simulink model "simu"  (R2023b)
settings: Solver=ode15s  StartTime=0.0  StopTime=20  RelTol=1e-4
values from neighbouring files (symbols this model uses):
  Bm = .015    (= 0.015)    [example_1.m]    (also in myStateTransitionFcn.m)
  g = 9.8    [example_1.m]    (also in myStateTransitionFcn.m)
  J = 4e-4    (= 0.0004)    [example_1.m]    (also in myStateTransitionFcn.m)
  Jl = 4e-4    (= 0.0004)    [example_1.m]    (also in myStateTransitionFcn.m)
  Jm = 4e-4    (= 0.0004)    [example_1.m]    (also in myStateTransitionFcn.m)
  k = .8    (= 0.8)    [example_1.m]    (also in myStateTransitionFcn.m)
  l = .3    (= 0.3)    [example_1.m]    (also in myStateTransitionFcn.m)
  m = .3    (= 0.3)    [example_1.m]    (also in myStateTransitionFcn.m)
  static_gain = inv(C*inv(-A+B*K)*B)    [example_1.m]
  x_est_initial = [pi/2;0;pi/2;0]    [example_1.m]
undefined symbols (not defined in the file or in its folder): beta, K
settings Model: Creator=Douglas  LastModifiedBy=Douglas

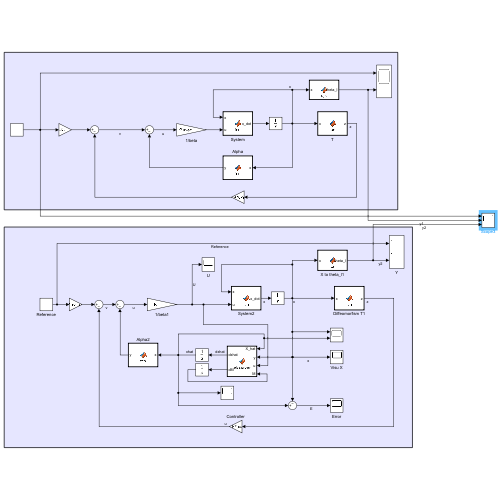
[thumbnail: Simulink's stored preview of the top-level diagram]
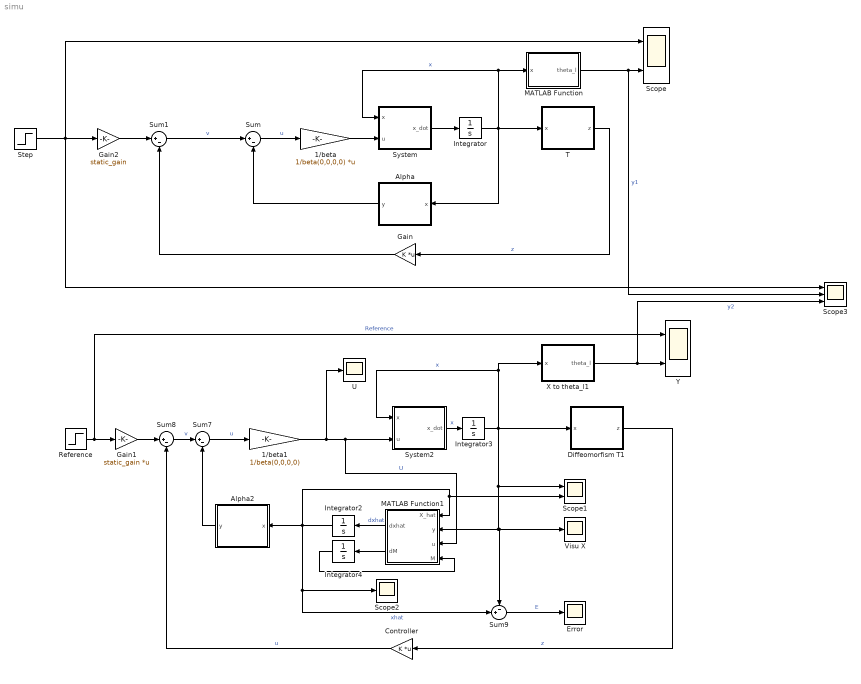
== system simu ==
  1/beta : Gain  Gain=1/beta(0,0,0,0)  Multiplication=Matrix(K*u) (u vector)
  1/beta1 : Gain  Gain=1/beta(0,0,0,0)
  Alpha : MATLAB Function  TreatAsAtomicUnit=on
  Alpha2 : MATLAB Function  TreatAsAtomicUnit=on
  Controller : Gain  Gain=K  Multiplication=Matrix(K*u) (u vector)
  Diffeomorfism T1 : MATLAB Function  TreatAsAtomicUnit=on
  Error : Scope
  Gain : Gain  Gain=K  Multiplication=Matrix(K*u) (u vector)
  Gain1 : Gain  Gain=static_gain  Multiplication=Matrix(K*u) (u vector)
  Gain2 : Gain  Gain=static_gain
  Integrator : Integrator  InitialCondition=x_est_initial
  Integrator2 : Integrator  InitialCondition=x_est_initial
  Integrator3 : Integrator  InitialCondition=x_est_initial
  Integrator4 : Integrator  InitialCondition=zeros(4,4)
  MATLAB Function : MATLAB Function  TreatAsAtomicUnit=on
  MATLAB Function1 : MATLAB Function  TreatAsAtomicUnit=on
  Reference : Step  Time=10  After=0.3  SampleTime=0
  Scope : Scope  NumInputPorts=2
  Scope1 : Scope  NumInputPorts=2
  Scope2 : Scope
  Scope3 : Scope  NumInputPorts=3
  Step : Step  Time=10  After=0.3  SampleTime=0
  Sum{,1,7..8} (4 alike) : Sum  Inputs=|+-
  Sum9 : Sum  Inputs=-+|
  System : MATLAB Function  TreatAsAtomicUnit=on
  System2 : MATLAB Function  TreatAsAtomicUnit=on
  T : MATLAB Function  TreatAsAtomicUnit=on
  U : Scope
  Visu X : Scope
  X to theta_l1 : MATLAB Function  TreatAsAtomicUnit=on
  Y : Scope  NumInputPorts=2
  wires:
  Sum1/1 -> Sum/1  "v"
  Sum/1 -> 1/beta/1  "u"
  1/beta/1 -> System/2(u)
  System/1(x_dot) -> Integrator/1
  Integrator/1 -> System/1(x), MATLAB Function/1(x), Alpha/1(x), T/1(x)  "x"
  Alpha/1(y) -> Sum/2
  Gain/1 -> Sum1/2
  T/1(z) -> Gain/1  "z"
  Gain2/1 -> Sum1/1
  Step/1 -> Scope3/1, Scope/1, Gain2/1
  MATLAB Function/1(theta_l) -> Scope3/2, Scope/2  "y1"
  Sum8/1 -> Sum7/1  "v"
  X to theta_l1/1(theta_l) -> Scope3/3, Y/2  "y2"
  MATLAB Function1/1(dxhat) -> Integrator2/1  "dxhat"
  Sum9/1 -> Error/1  "E"
  Diffeomorfism T1/1(z) -> Controller/1  "z"
  Integrator3/1 -> Visu X/1, Sum9/1, MATLAB Function1/2(y), Scope1/1, X to theta_l1/1(x), System2/1(x), Diffeomorfism T1/1(x)  "x"
  Alpha2/1(y) -> Sum7/2
  Sum7/1 -> 1/beta1/1  "u"
  Integrator2/1 -> Scope2/1, Sum9/2, Scope1/2, MATLAB Function1/1(X_hat), Alpha2/1(x)  "xhat"
  Reference/1 -> Gain1/1, Y/1  "Reference"
  Gain1/1 -> Sum8/1
  1/beta1/1 -> MATLAB Function1/3(u), System2/2(u), U/1  "U"
  System2/1(x_dot) -> Integrator3/1  "x"
  MATLAB Function1/2(dM) -> Integrator4/1
  Integrator4/1 -> MATLAB Function1/4(M)
  Controller/1 -> Sum8/2  "u"

== matlab function simu/X to theta_l1 ==
  data: x input; theta_l output
function theta_l = fcn(x)



theta_l = (pi/2) - x(1);

== matlab function simu/MATLAB Function1 ==
  data: X_hat input; y input; u input; dxhat output; dM output; M input; J parameter; k parameter; Bm parameter; m parameter; l parameter; g parameter
function [dxhat, dM] = observer(X_hat, y, u, M, J, k, Bm, m, l, g)
A = [0 1 0 0; (-(1/J)*k + (1/J)*m*g*l*sin(X_hat(1))) 0 ((1/J)*k) 0; 0 0 0 1; (k/J) 0 -(k/J) -(Bm/J)];
B = [0;0;0;1/J];
C = [-1 0 0 0];
D = 0;

V = diag([1e4 1e4 1e4 1e4]);
W = 1e-5;

dxhat = [ X_hat(2);
            -1/J*(k*(X_hat(1)-X_hat(3)) + m*g*l*cos(X_hat(1)));
            X_hat(4);
            1/J*(-Bm*X_hat(4) + k*(X_hat(1)-X_hat(3)) + u)] -  M*C'*inv(W)*(X_hat(1) - y(1));

dM = A*M + M*A' - M*C'*inv(W)*C*M + V;

== matlab function simu/Alpha ==
  data: x input; y output
function y = fcn(x)
alpha = @(x1,x2,x3,x4)x1.*-4.0e+6+x3.*4.0e+6+x4.*7.5e+4-x2.^2.*cos(x1).*2.205e+3+(sin(x1).*2.205e+3-2.0e+3).*(x1.*2.0e+3-x3.*2.0e+3+cos(x1).*2.205e+3);
y = alpha(x(1),x(2),x(3),x(4));

== matlab function simu/System ==
  data: x input; u input; x_dot output; k parameter; Jm parameter; Jl parameter; m parameter; g parameter; l parameter; Bm parameter
function x_dot = fcn(x, u, k, Jm, Jl, m, g, l, Bm)

x1 = x(1);
x2 = x(2);
x3 = x(3);
x4 = x(4);

x1_dot = x2;
x2_dot = (-1/Jl)*(k*(x1-x3) + m*g*l*cos(x1));
x3_dot = x4;
x4_dot = (-Bm/Jm)*x4 + (k/Jm)*(x1-x3) + (1/Jm)*u;

x_dot = [x1_dot;x2_dot; x3_dot; x4_dot];

== matlab function simu/T ==
  data: x input; z output
function z = fcn(x)
diffeo = @(x1,x2,x3,x4)[-x1+pi./2.0,-x2,x1.*2.0e+3-x3.*2.0e+3+cos(x1).*2.205e+3,x4.*-2.0e+3-x2.*(sin(x1).*2.205e+3-2.0e+3)];

z = diffeo(x(1),x(2),x(3), x(4));

== matlab function simu/MATLAB Function ==
  data: x input; theta_l output
function theta_l = fcn(x)



theta_l = (pi/2) - x(1);

== matlab function simu/Alpha2 ==
  data: x input; y output
function y = fcn(x)
alpha = @(x1,x2,x3,x4)x1.*-4.0e+6+x3.*4.0e+6+x4.*7.5e+4-x2.^2.*cos(x1).*2.205e+3+(sin(x1).*2.205e+3-2.0e+3).*(x1.*2.0e+3-x3.*2.0e+3+cos(x1).*2.205e+3);
y = alpha(x(1),x(2),x(3),x(4));

== matlab function simu/Diffeomorfism T1 ==
  data: x input; z output
function z = fcn(x)
diffeo = @(x1,x2,x3,x4)[-x1+pi./2.0,-x2,x1.*2.0e+3-x3.*2.0e+3+cos(x1).*2.205e+3,x4.*-2.0e+3-x2.*(sin(x1).*2.205e+3-2.0e+3)];

z = diffeo(x(1),x(2),x(3), x(4));

== matlab function simu/System2 ==
  data: x input; u input; x_dot output; k parameter; Jm parameter; Jl parameter; m parameter; g parameter; l parameter; Bm parameter
function x_dot = fcn(x, u, k, Jm, Jl, m, g, l, Bm)

x1 = x(1);
x2 = x(2);
x3 = x(3);
x4 = x(4);

x1_dot = x2;
x2_dot = (-1/Jl)*(k*(x1-x3) + m*g*l*cos(x1));
x3_dot = x4;
x4_dot = (-Bm/Jm)*x4 + (k/Jm)*(x1-x3) + (1/Jm)*u;

x_dot = [x1_dot;x2_dot; x3_dot; x4_dot];
